simulink model "untitled"  (R2019a)
settings: Solver=FixedStepDiscrete  StartTime=0.0  StopTime=10.0  RelTol=1e-3
undefined symbols (not defined in the file): darwinop_communication_setup
settings Model: Creator=vasi_ko  LastModifiedBy=vasi_ko
settings OptimizationCC: DefaultParameterBehavior=Inlined  EnhancedBackFolding=on  PassReuseOutputArgsAs=Individual arguments  OptimizeBlockOrder=speed  DifferentSizesBufferReuse=on  OptimizationCustomize=off
settings DebuggingCC: ParameterTunabilityLossMsg=error
settings HardwareCC: ProdBitPerPointer=32  ProdBitPerSizeT=32  ProdBitPerPtrDiffT=32  ProdLargestAtomicFloat=None  ProdIntDivRoundTo=Undefined  ProdWordSize=32  ProdHWDeviceType=Generic->32-bit Embedded Processor
settings SFSimCC: MATLABDynamicMemAlloc=off
settings RTWCC: SystemTargetFile=darwinoplib.tlc  GenCodeOnly=on  TemplateMakefile=darwinoplib.tmf  Description=DarwinOP code generator  IncludeHyperlinkInReport=on  TargetLang=C++
settings CodeAppCC: ForceParamTrailComments=on  IgnoreCustomStorageClasses=off  OperatorAnnotations=on  SimulinkDataObjDesc=on  SFDataObjDesc=on  InsertBlockDesc=on
settings STFCustomTargetCC: TargetLangStandard=C++03 (ISO)  MultiwordLength=256  CombineOutputUpdateFcns=on  ERTCustomFileBanners=on  SupportContinuousTime=off  SupportNonInlinedSFcns=off  RemoveResetFunc=on  MATLABClassNameForMDSCustomization=Simulink.SoftwareTarget.ERTCustomization  GRTInterface=off  SystemTargetFile=darwinoplib.tlc
settings ERTTargetCC: TargetLangStandard=C++03 (ISO)  ParMdlRefBuildCompliant=off  CompOptLevelCompliant=off  ConcurrentExecutionCompliant=off  ModelStepFunctionPrototypeControlCompliant=off  CPPClassGenCompliant=off  UseToolchainInfoCompliant=off  InlinedParameterPlacement=NonHierarchical  ERTCustomFileTemplate=darwinoplib_main.tlc

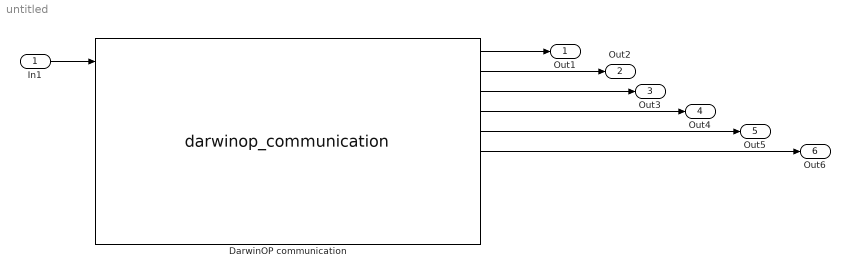
== system untitled ==
  In1 : Inport
  DarwinOP communication : M-S-Function  StartFcn=darwinop_communication_setup('StartFcn');  StopFcn=darwinop_communication_setup('StopFcn');  FunctionName=darwinop_communication  Parameters=IP,Port,Protocol,SampleTime,Frame,ReadIndex,WriteIndex  mask{IP=192.168.123.1, Port=1234, Protocol=tcp, SampleTime=0.5, Frame=[ 2 1 30 2 3 1 6 2 0 0 2 2 15 1 2 7 32 2 2 7 36 6 3 7 24 1 0 3 7 26 1 0 3 7 32 2 0 0 3 7 73 1 0 2 200 44 6 2 112 25 1], ReadIndex=[ 1 2;3 1;4 2;6 2;8 2;10 2;12 2;14 2;16 2;18 1], WriteIndex=[ 9 2;27 1;32 1;37 2;43 1]}
      settings: DeleteFcn=darwinop_communication_setup('DeleteFcn');  ModelCloseFcn=darwinop_communication_setup('ModelCloseFcn');  NameChangeFcn=darwinop_communication_setup('NameChangeFcn');  OpenFcn=darwinop_communication_setup('OpenFcn');
      mask TypeOptions Protocol: tcp | udp
      mask Display:
      | image('darwin-blk.jpg')
      | 
      | port_label('output',1,'Right Shoulder Pitch(1)/Goal Position')
      | port_label('output',2,'Left Shoulder Pitch(2)/Max Torque (H)')
      | port_label('output',3,'Right Hip Yaw(7)/Moving Speed')
      | port_label('output',4,'Right Hip Yaw(7)/Position')
      | port_label('output',5,'Right Hip Yaw(7)/Speed')
      | port_label('output',6,'Right Hip Yaw(7)/Load')
      | port_label('output',7,'Sub controller(200)/ACC X')
      | port_label('output',8,'Sub controller(200)/ACC Y')
      | port_label('output',9,'Sub controller(200)/ACC Z')
      | port_label('output',10,'Left Foot(112)/LED')
      | 
      | port_label('input',1,'Right Shoulder Pitch(1)/CW Angle Limit')
      | port_label('input',2,'Right Hip Yaw(7)/Torque Enable')
      | port_label('input',3,'Right Hip Yaw(7)/D Gain')
      | port_label('input',4,'Right Hip Yaw(7)/Moving Speed')
      | port_label('input',5,'Right Hip Yaw(7)/Goal Acceleration')
  Out1 : Outport
  Out2 : Outport  Port=2
  Out3 : Outport  Port=3
  Out4 : Outport  Port=4
  Out5 : Outport  Port=5
  Out6 : Outport  Port=6
  wires:
  In1/1 -> DarwinOP communication/1
  DarwinOP communication/1 -> Out1/1
  DarwinOP communication/2 -> Out2/1
  DarwinOP communication/3 -> Out3/1
  DarwinOP communication/4 -> Out4/1
  DarwinOP communication/5 -> Out5/1
  DarwinOP communication/6 -> Out6/1
